simulink model "asinx2model"  (Simulink 8.6)
settings: Solver=ode45  StartTime=0.0  StopTime=10.0  RelTol=1e-3
values from neighbouring files (symbols this model uses):
  a = 1    [Prelims.m]    (also in Prelims_no_b4m.m; Simulation1.mat)
  K_lqr = lqr(A,B,Q,R,[])    [Prelims.m]    (also in Prelims_no_b4m.m; Simulation1.mat = [1 1.73205080757])
  u_max = 1.2    [Prelims.m]    (also in Prelims_no_b4m.m = 2.75; Simulation1.mat = 2.75)
  u_min = -1.2    [Prelims.m]    (also in Prelims_no_b4m.m = -2.75; Simulation1.mat = -2.75)
  x1_0 = pi/2    (= 1.57079632679)    [Prelims.m]    (also in Prelims_no_b4m.m; Simulation1.mat)
  x2_0 = pi/4    (= 0.785398163397)    [Prelims.m]    (also in Prelims_no_b4m.m; Simulation1.mat)
settings Model: Creator=mLab  LastModifiedBy=mlab-retro
settings DebuggingCC: FcnCallInpInsideContextMsg=EnableAllAsWarning
settings GRTTargetCC: CombineOutputUpdateFcns=on  GRTInterface=off

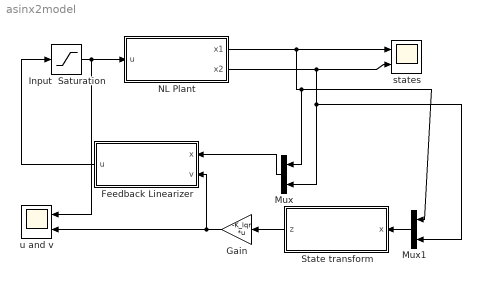
== system asinx2model ==
  Feedback Linearizer : Subsystem
  Gain : Gain  Gain=-K_lqr  Multiplication=Matrix(K*u) (u vector)
  Input  Saturation : Saturate  UpperLimit=u_max  LowerLimit=u_min
  Mux : Mux  Inputs=2
  Mux1 : Mux  Inputs=2
  NL Plant : Subsystem
  State transform : Subsystem
  states : Scope  NumInputPorts=2
  u and v : Scope  NumInputPorts=2
  wires:
  NL Plant/1(x1) -> states/1, Mux/1, Mux1/1
  NL Plant/2(x2) -> states/2, Mux/2, Mux1/2
  Mux/1 -> Feedback Linearizer/1(x)
  Mux1/1 -> State transform/1(x)
  State transform/1(z) -> Gain/1
  Gain/1 -> Feedback Linearizer/2(v), u and v/2
  Feedback Linearizer/1(u) -> Input  Saturation/1
  Input  Saturation/1 -> NL Plant/1(u), u and v/1

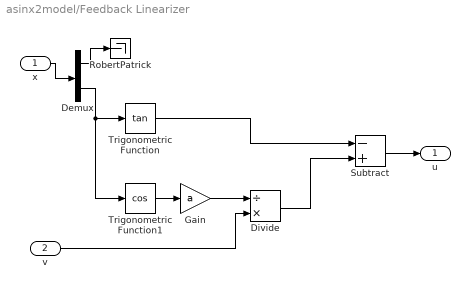
== system asinx2model/Feedback Linearizer ==
  x : Inport
  v : Inport  Port=2
  Demux : Demux  Outputs=2
  Divide : Product  Inputs=/*
  Gain : Gain  Gain=a
  RobertPatrick : Terminator
  Subtract : Sum  Inputs=-+
  Trigonometric Function : Trigonometry  Operator=tan
  Trigonometric Function1 : Trigonometry  Operator=cos
  u : Outport
  wires:
  x/1 -> Demux/1
  Demux/1 -> RobertPatrick/1
  Demux/2 -> Trigonometric Function/1, Trigonometric Function1/1
  Trigonometric Function1/1 -> Gain/1
  Gain/1 -> Divide/1
  Subtract/1 -> u/1
  Trigonometric Function/1 -> Subtract/1
  Divide/1 -> Subtract/2
  v/1 -> Divide/2

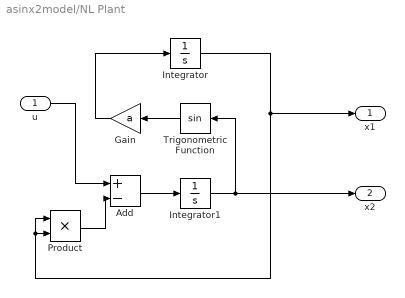
== system asinx2model/NL Plant ==
  u : Inport
  Add : Sum  Inputs=+-
  Gain : Gain  Gain=a
  Integrator : Integrator  InitialCondition=x1_0
  Integrator1 : Integrator  InitialCondition=x2_0
  Product : Product  RndMeth=Zero
  Trigonometric Function : Trigonometry
  x1 : Outport
  x2 : Outport  Port=2
  wires:
  Trigonometric Function/1 -> Gain/1
  Gain/1 -> Integrator/1
  Integrator/1 -> x1/1, Product/2, Product/1
  Integrator1/1 -> Trigonometric Function/1, x2/1
  Add/1 -> Integrator1/1
  Product/1 -> Add/2
  u/1 -> Add/1

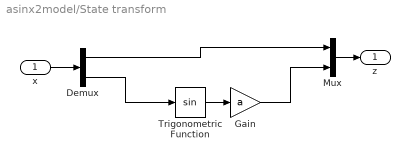
== system asinx2model/State transform ==
  x : Inport
  Demux : Demux  Outputs=2
  Gain : Gain  Gain=a
  Mux : Mux  Inputs=2
  Trigonometric Function : Trigonometry
  z : Outport
  wires:
  Trigonometric Function/1 -> Gain/1
  x/1 -> Demux/1
  Demux/2 -> Trigonometric Function/1
  Mux/1 -> z/1
  Gain/1 -> Mux/2
  Demux/1 -> Mux/1
